simulink model "problem1c"  (Simulink 8.7)
settings: Solver=VariableStepAuto  StartTime=0.0  StopTime=5  RelTol=1e-3
libraries: simulink x1
settings Model: Creator=asus1  LastModifiedBy=asus1
settings DataIOCC: LimitDataPoints=off  SaveFormat=Dataset
settings DebuggingCC: UnderspecifiedInitializationDetection=Simplified  MergeDetectMultiDrivingBlocksExec=error
settings HardwareCC: ProdBitPerPointer=64  ProdLargestAtomicFloat=Float  ProdIntDivRoundTo=Zero  ProdEndianess=LittleEndian  ProdWordSize=64  ProdHWDeviceType=Intel->x86-64 (Windows64)
settings ModelReferenceCC: PropagateSignalLabelsOutOfModel=on
settings ConfigComp: CovModelRefEnable=off

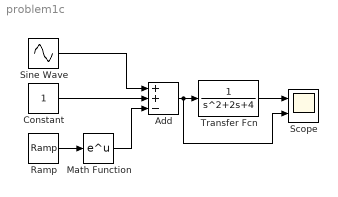
== system problem1c ==
  Add : Sum  Inputs=++-
  Constant : Constant
  Math Function : Math  SaturateOnIntegerOverflow=on
  Ramp : simulink/Sources/Ramp  slope=-0.5  start=0  X0=0
  Scope : Scope  NumInputPorts=2
  Sine Wave : Sin  Amplitude=5  SampleTime=0
  Transfer Fcn : TransferFcn  Numerator=[0 0 1]  Denominator=[1 2 4]
  wires:
  Constant/1 -> Add/2
  Sine Wave/1 -> Add/1
  Ramp/1 -> Math Function/1
  Math Function/1 -> Add/3
  Transfer Fcn/1 -> Scope/1
  Add/1 -> Scope/2, Transfer Fcn/1
